simulink model "QCM_project"  (R2021a)
settings: Solver=VariableStepAuto  StartTime=0.0  StopTime=20  RelTol=1e-3
undefined symbols (not defined in the file): c_com, c_re, k1, k2, mc, ms, v
settings Model: Creator=sampa  LastModifiedBy=sampa

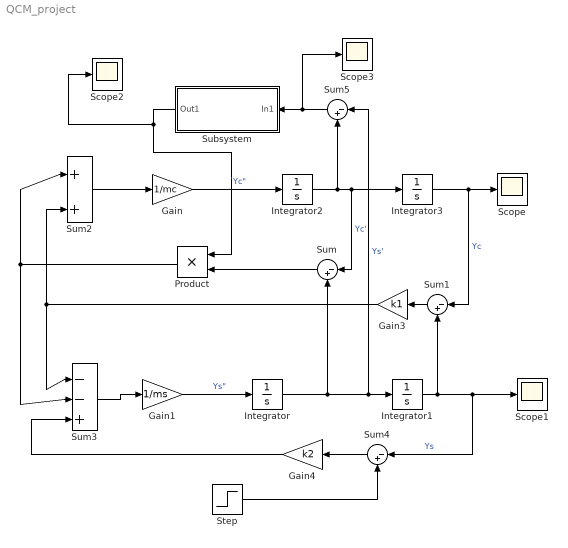
== system QCM_project ==
  Gain : Gain  Gain=1/mc
  Gain1 : Gain  Gain=1/ms
  Gain3 : Gain  Gain=k1
  Gain4 : Gain  Gain=k2
  Integrator{,1..3} (4 alike) : Integrator
  Product : Product
  Scope{,1..3} (4 alike) : Scope
  Step : Step  After=5  SampleTime=0
  Subsystem : Subsystem
  Sum{,1,4..5} (4 alike) : Sum  Inputs=|-+
  Sum2 : Sum  Inputs=|++
  Sum3 : Sum  Inputs=|--+
  wires:
  Gain/1 -> Integrator2/1  "Yc\""
  Integrator2/1 -> Sum5/2, Integrator3/1, Sum/1  "Yc'"
  Integrator3/1 -> Sum1/1, Scope/1  "Yc"
  Integrator/1 -> Integrator1/1, Sum5/1, Sum/2  "Ys'"
  Gain1/1 -> Integrator/1  "Ys\""
  Integrator1/1 -> Sum4/1, Scope1/1, Sum1/2  "Ys"
  Sum/1 -> Product/2
  Sum1/1 -> Gain3/1
  Sum2/1 -> Gain/1
  Sum3/1 -> Gain1/1
  Sum4/1 -> Gain4/1
  Gain4/1 -> Sum3/3
  Step/1 -> Sum4/2
  Sum5/1 -> Scope3/1, Subsystem/1(In1)
  Subsystem/1(Out1) -> Scope2/1, Product/1
  Product/1 -> Sum3/2, Sum2/1
  Gain3/1 -> Sum2/2, Sum3/1

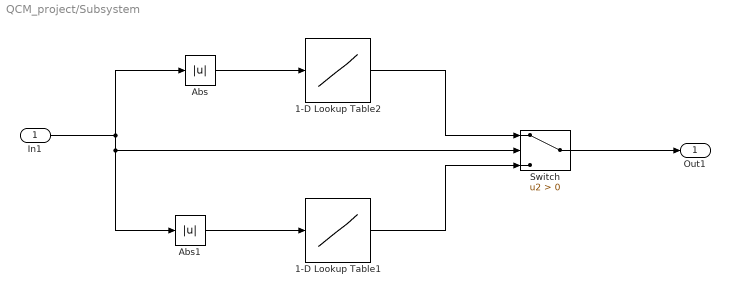
== system QCM_project/Subsystem ==
  In1 : Inport
  1-D Lookup Table1 : Lookup_n-D  NumberOfTableDimensions=1  BreakpointsForDimension1=v  Table=c_re  InternalRulePriority=Speed  RndMeth=Simplest  InputSameDT=on
  1-D Lookup Table2 : Lookup_n-D  NumberOfTableDimensions=1  BreakpointsForDimension1=v  Table=c_com  InternalRulePriority=Speed  RndMeth=Simplest  InputSameDT=on
  Abs : Abs
  Abs1 : Abs
  Switch : Switch  Criteria=u2 > Threshold
  Out1 : Outport
  wires:
  Abs/1 -> 1-D Lookup Table2/1
  Abs1/1 -> 1-D Lookup Table1/1
  In1/1 -> Switch/2, Abs1/1, Abs/1
  1-D Lookup Table2/1 -> Switch/1
  1-D Lookup Table1/1 -> Switch/3
  Switch/1 -> Out1/1
